simulink model "sampleModel1433_3"  (R2023a)
settings: Solver=VariableStepAuto  StartTime=0.0  StopTime=10.0  RelTol=1e-3
libraries: hdlsllib x7, simulink x2
settings Model: Creator=user1  LastModifiedBy=user1

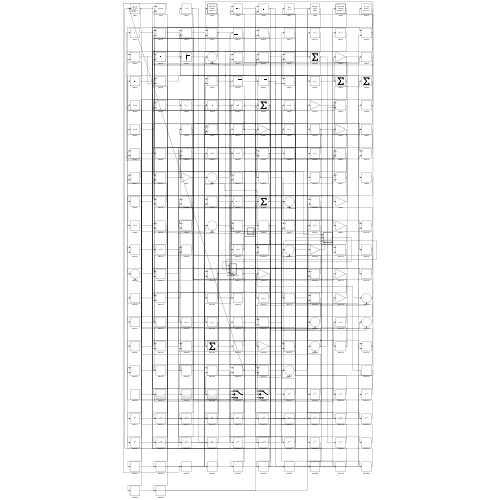
[thumbnail: Simulink's stored preview of the top-level diagram]
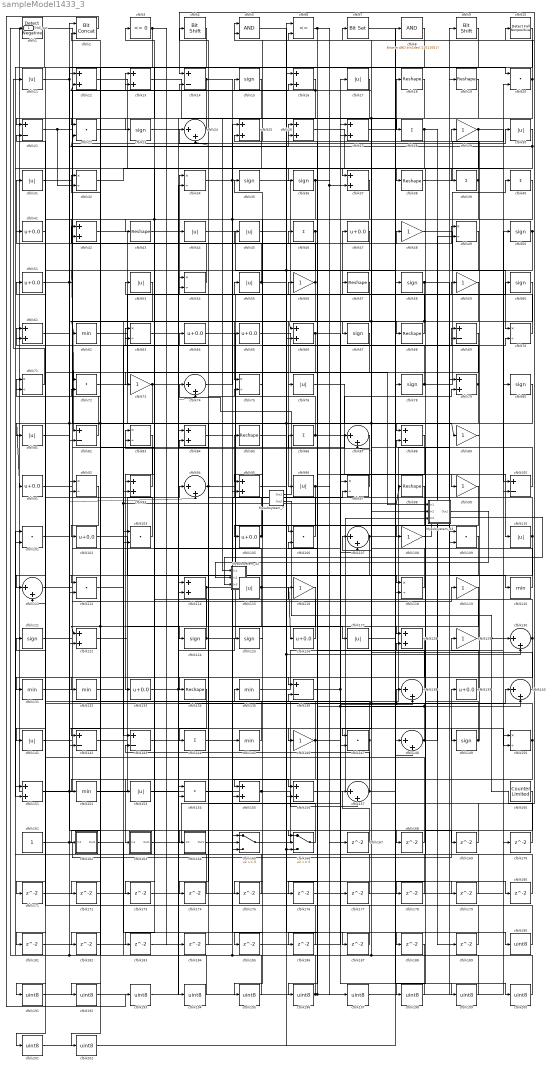
== system sampleModel1433_3 ==
  Mysubsystem_42 : Subsystem  TreatAsAtomicUnit=on  RTWFcnName=Mysubsystem_42
      settings: RTWFcnNameOpts=User specified  RTWFileNameOpts=Use function name
  Mysubsystem_43 : Subsystem  TreatAsAtomicUnit=on  RTWFcnName=Mysubsystem_43
      settings: RTWFcnNameOpts=User specified  RTWFileNameOpts=Use function name
  Mysubsystem_7 : Subsystem  TreatAsAtomicUnit=on  RTWFcnName=Mysubsystem_7
      settings: RTWFcnNameOpts=User specified  RTWFileNameOpts=Use function name
  cfblk1 : hdlsllib/Logic and Bit Operations/Detect Fall Negative  vinit=0  OutDataTypeStr=uint8
  cfblk10 : hdlsllib/Logic and Bit Operations/Detect Fall Nonpositive  vinit=0  OutDataTypeStr=uint8
  cfblk{14,21,69,82,100,136,142..143} (8 alike) : Sum  Inputs=+-  OutDataTypeStr=uint8
  cfblk{20,22,72,101,103,106,109,112,147,154} (10 alike) : DotProduct  OutDataTypeStr=uint8
  cfblk{41,47,51,64..65,91,102,105,126,133,139} (11 alike) : Bias  Bias=0.0  SaturateOnIntegerOverflow=off
  cfblk{24,74,87,94,107,111,130,138,140,148,157} (11 alike) : Sum  Inputs=|++  OutDataTypeStr=uint8
  cfblk{29,48,56,59,73,89,99,108,116,119,129,146} (12 alike) : Gain  OutDataTypeStr=uint8
  cfblk{11,17,30..31,44..45,53,55,76,81,96,110,115,127,141,153} (16 alike) : Abs  OutDataTypeStr=uint8  SaturateOnIntegerOverflow=off
  cfblk{12..13,16,25..27,37,42,61,66,79,84,88,93,95,114,122,128,151,155..156} (21 alike) : Sum  OutDataTypeStr=uint8
  cfblk{32,34,49,54,63,70..71,75,83,92,97,118,150} (13 alike) : Product  Inputs=*/  OutDataTypeStr=uint8  RndMeth=Zero  SaturateOnIntegerOverflow=on
  cfblk{62,120,131..132,135,145,152} (7 alike) : MinMax  OutDataTypeStr=uint8
  cfblk{15,23,35..36,50,58,60,67,78,80,121,124..125,149} (14 alike) : Signum
  cfblk{18..19,38,43,57,68,85,98,134} (9 alike) : Reshape
  cfblk{28,39..40,46,86,144} (6 alike) : Sum  Inputs=+  OutDataTypeStr=uint8
  cfblk160 : hdlsllib/Sources/Counter Limited  uplimit=7  tsamp=-1
  cfblk161 : Constant  OutDataTypeStr=uint8  SampleTime=-1
  cfblk162 : Subsystem
      settings: LibrarySourceBlock=|
      | hdlsllib/Ports &
      | Subsystems/Subsystem
  cfblk163 : Subsystem
      settings: LibrarySourceBlock=|
      | hdlsllib/Ports &
      | Subsystems/Subsystem
  cfblk164 : Subsystem
      settings: LibrarySourceBlock=|
      | hdlsllib/Ports &
      | Subsystems/Subsystem
  cfblk165 : Switch  OutDataTypeStr=uint8  SaturateOnIntegerOverflow=off  InputSameDT=off
  cfblk166 : Switch  OutDataTypeStr=uint8  SaturateOnIntegerOverflow=off  InputSameDT=off
  cfblk{167..189} (23 alike) : Delay  SampleTime=1
  cfblk{190..202} (13 alike) : DataTypeConversion  OutDataTypeStr=uint8  SaturateOnIntegerOverflow=off  RndMeth=Floor
  cfblk2 : hdlsllib/Logic and Bit Operations/Bit Concat  numInputs=2
  cfblk3 : hdlsllib/Logic and Bit Operations/Compare To Zero  relop=<=  OutDataTypeStr=uint8
  cfblk4 : hdlsllib/Logic and Bit Operations/Bit Shift  mode=Shift Left Logical  N=0
  cfblk5 : Logic  AllPortsSameDT=off  OutDataTypeStr=boolean
  cfblk6 : RelationalOperator  Operator=<=  OutDataTypeStr=boolean  InputSameDT=off
  cfblk7 : simulink/Logic and Bit Operations/Bit Set  iBit=0
      settings: LibrarySourceBlock=|
      | hdlsllib/Logic and Bit
      | Operations/Bit Set
  cfblk8 : simulink/Logic and Bit Operations/Bitwise Operator  logicop=AND  UseBitMask=on  BitMask=bin2dec('11011001')  BitMaskRealWorld=Stored Integer
      settings: LibrarySourceBlock=|
      | hdlsllib/Logic and Bit
      | Operations/Bitwise
      | Operator
  cfblk9 : hdlsllib/Logic and Bit Operations/Bit Shift  mode=Shift Left Logical  N=0
  Hdl_out : Outport  OutDataTypeStr=uint8
  wires:
  cfblk105/1 -> cfblk61/1, cfblk75/2
  cfblk73/1 -> cfblk91/1, cfblk172/1, cfblk60/1
  cfblk71/1 -> cfblk11/1
  cfblk145/1 -> cfblk135/1
  cfblk115/1 -> cfblk126/1, cfblk63/2, cfblk174/1
  cfblk131/1 -> cfblk48/1
  cfblk133/1 -> cfblk74/2, cfblk169/1
  cfblk54/1 -> cfblk34/1
  cfblk152/1 -> cfblk94/1
  cfblk86/1 -> cfblk110/1, cfblk54/2
  cfblk1/1 -> cfblk88/1, cfblk101/2
  cfblk31/1 -> cfblk16/2
  cfblk89/1 -> cfblk29/1
  cfblk6/1 -> cfblk37/2, cfblk167/1, cfblk106/1
  cfblk135/1 -> cfblk50/1
  cfblk60/1 -> cfblk96/1
  cfblk118/1 -> cfblk55/1
  cfblk42/1 -> cfblk76/1
  cfblk161/1 -> cfblk139/1, cfblk94/2
  cfblk74/1 -> cfblk25/1
  cfblk49/1 -> cfblk141/1
  cfblk51/1 -> cfblk15/1, cfblk65/1
  cfblk68/1 -> cfblk66/1, cfblk3/1
  cfblk45/1 -> cfblk130/2, cfblk188/1
  cfblk120/1 -> cfblk53/1
  cfblk24/1 -> cfblk21/1
  cfblk35/1 -> cfblk68/1
  cfblk157/1 -> cfblk13/1, cfblk69/2
  cfblk12/1 -> cfblk100/1
  cfblk78/1 -> cfblk40/1, cfblk45/1
  cfblk8/1 -> cfblk202/1
  cfblk160/1 -> cfblk198/1
  cfblk26/1 -> cfblk38/1
  cfblk163/1(Out1) -> cfblk17/1
  cfblk121/1 -> cfblk119/1
  cfblk126/1 -> cfblk83/1
  cfblk141/1 -> cfblk30/1
  cfblk4/1 -> cfblk111/1
  cfblk83/1 -> cfblk133/1
  cfblk25/1 -> cfblk43/1
  cfblk79/1 -> cfblk122/2, cfblk111/2, cfblk26/1
  cfblk124/1 -> cfblk47/1, cfblk42/2
  cfblk96/1 -> cfblk156/2, cfblk177/1
  cfblk37/1 -> cfblk82/1, cfblk73/1, cfblk95/2
  cfblk107/1 -> cfblk115/1, cfblk150/2
  cfblk155/1 -> cfblk157/2, Hdl_out/1
  cfblk20/1 -> Mysubsystem_42/1(In1), cfblk5/1
  cfblk130/1 -> cfblk132/1, cfblk63/1
  cfblk22/1 -> cfblk58/1
  cfblk9/1 -> cfblk23/1
  cfblk50/1 -> cfblk72/1, cfblk166/2, cfblk10/1
  cfblk91/1 -> cfblk79/2
  cfblk103/1 -> cfblk51/1
  cfblk142/1 -> cfblk9/1
  cfblk30/1 -> cfblk128/1, cfblk22/2
  cfblk58/1 -> cfblk62/1, cfblk87/2, cfblk120/1
  cfblk72/1 -> cfblk27/2
  cfblk44/1 -> cfblk78/1
  cfblk18/1 -> cfblk67/1, cfblk36/1
  cfblk27/1 -> cfblk18/1
  cfblk138/1 -> cfblk46/1
  cfblk88/1 -> cfblk136/1
  cfblk153/1 -> cfblk140/1
  cfblk21/1 -> cfblk143/1, cfblk32/2
  cfblk82/1 -> cfblk71/1
  cfblk147/1 -> cfblk4/1, cfblk182/1
  cfblk102/1 -> cfblk148/2
  cfblk165/1 -> cfblk87/1
  cfblk140/1 -> cfblk107/1
  cfblk64/1 -> cfblk118/1
  cfblk19/1 -> cfblk196/1
  cfblk56/1 -> cfblk31/1, cfblk142/1
  cfblk16/1 -> cfblk12/2, cfblk112/2
  cfblk13/1 -> cfblk28/1
  cfblk92/1 -> cfblk102/1
  cfblk129/1 -> cfblk24/1
  cfblk139/1 -> cfblk129/1
  cfblk40/1 -> cfblk105/1
  cfblk134/1 -> cfblk144/1
  cfblk66/1 -> cfblk99/1, cfblk81/1
  cfblk10/1 -> cfblk82/2
  cfblk106/1 -> cfblk35/1
  cfblk94/1 -> cfblk24/2, cfblk147/2
  cfblk164/1(Out1) -> cfblk97/2
  cfblk136/1 -> cfblk140/2, cfblk199/1, cfblk70/2
  cfblk122/1 -> cfblk124/1
  cfblk101/1 -> cfblk164/1(In1)
  cfblk23/1 -> cfblk66/2
  cfblk39/1 -> cfblk5/2, cfblk181/1
  cfblk61/1 -> cfblk146/1
  cfblk149/1 -> cfblk59/1, cfblk128/2
  cfblk93/1 -> cfblk42/1
  cfblk62/1 -> cfblk107/2
  cfblk34/1 -> cfblk127/1, cfblk39/1
  cfblk111/1 -> cfblk49/1
  cfblk3/1 -> cfblk184/1, cfblk192/1
  cfblk47/1 -> cfblk93/1
  cfblk84/1 -> cfblk145/1
  cfblk100/1 -> cfblk6/2
  cfblk53/1 -> cfblk93/2
  cfblk76/1 -> cfblk109/1
  cfblk11/1 -> cfblk20/1, cfblk165/3
  cfblk15/1 -> cfblk114/2
  cfblk48/1 -> cfblk70/1
  cfblk143/1 -> cfblk125/1
  cfblk17/1 -> cfblk92/2
  cfblk46/1 -> cfblk153/1, cfblk186/1
  cfblk70/1 -> cfblk44/1
  cfblk14/1 -> cfblk118/2, cfblk22/1
  cfblk55/1 -> cfblk89/1, cfblk179/1, cfblk32/1
  cfblk81/1 -> cfblk14/2
  cfblk36/1 -> cfblk131/1, cfblk197/1
  cfblk144/1 -> cfblk166/1
  cfblk95/1 -> cfblk108/1
  cfblk166/1 -> cfblk54/1
  cfblk7/1 -> cfblk200/1
  cfblk38/1 -> cfblk20/2
  cfblk148/1 -> cfblk56/1, cfblk138/1, cfblk116/1, cfblk49/2
  cfblk43/1 -> cfblk149/1
  cfblk112/1 -> cfblk86/1, cfblk98/1
  cfblk150/1 -> Mysubsystem_43/2(In2), cfblk121/1, cfblk175/1
  cfblk87/1 -> cfblk83/2
  cfblk110/1 -> cfblk85/1, cfblk142/2
  cfblk97/1 -> cfblk64/1
  cfblk28/1 -> cfblk151/2, cfblk189/1
  cfblk146/1 -> cfblk163/1(In1), cfblk41/1, cfblk138/2
  cfblk125/1 -> cfblk155/1
  cfblk151/1 -> cfblk84/1, cfblk26/2
  cfblk59/1 -> cfblk75/1
  cfblk116/1 -> cfblk122/1, cfblk162/1(In1)
  cfblk85/1 -> cfblk109/2
  cfblk32/1 -> cfblk37/1
  cfblk57/1 -> cfblk112/1
  cfblk29/1 -> cfblk80/1, cfblk183/1
  cfblk80/1 -> cfblk134/1, cfblk147/1
  cfblk132/1 -> cfblk69/1
  cfblk67/1 -> cfblk95/1
  cfblk114/1 -> cfblk152/1, cfblk156/1
  cfblk167/1 -> cfblk157/1
  cfblk5/1 -> cfblk168/1
  cfblk168/1 -> cfblk71/2
  cfblk169/1 -> cfblk16/1
  cfblk170/1 -> cfblk25/2
  cfblk128/1 -> cfblk171/1
  cfblk171/1 -> cfblk165/1
  cfblk172/1 -> cfblk148/1
  cfblk109/1 -> cfblk173/1
  cfblk173/1 -> cfblk79/1
  cfblk174/1 -> cfblk13/2
  cfblk175/1 -> cfblk151/1
  cfblk119/1 -> cfblk176/1
  cfblk176/1 -> cfblk100/2
  cfblk177/1 -> cfblk114/1
  cfblk99/1 -> cfblk178/1
  cfblk178/1 -> cfblk61/2
  cfblk179/1 -> cfblk143/2
  cfblk127/1 -> cfblk180/1
  cfblk180/1 -> cfblk88/2
  cfblk181/1 -> cfblk34/2
  cfblk182/1 -> cfblk103/2
  cfblk183/1 -> cfblk155/2
  cfblk184/1 -> cfblk84/2
  cfblk98/1 -> cfblk185/1
  cfblk185/1 -> cfblk27/1
  cfblk186/1 -> cfblk72/2
  cfblk162/1(Out1) -> cfblk187/1
  cfblk187/1 -> cfblk136/2
  cfblk188/1 -> cfblk1/1
  cfblk189/1 -> cfblk21/2
  cfblk154/1 -> cfblk190/1
  cfblk190/1 -> cfblk97/1
  cfblk69/1 -> cfblk191/1
  cfblk191/1 -> cfblk154/1
  cfblk192/1 -> cfblk154/2
  cfblk2/1 -> cfblk193/1
  cfblk193/1 -> cfblk170/1
  cfblk63/1 -> cfblk194/1
  cfblk194/1 -> cfblk2/1
  cfblk75/1 -> cfblk195/1
  cfblk195/1 -> cfblk2/2
  cfblk196/1 -> cfblk106/2, cfblk150/1, cfblk165/2, cfblk92/1
  cfblk197/1 -> cfblk19/1
  cfblk198/1 -> cfblk101/1, cfblk12/1
  cfblk199/1 -> cfblk7/1
  cfblk200/1 -> cfblk57/1, cfblk103/1
  cfblk41/1 -> cfblk201/1
  cfblk201/1 -> cfblk8/1
  cfblk202/1 -> cfblk166/3, cfblk6/1
  Mysubsystem_7/2(Out2) -> cfblk14/1, cfblk130/1
  Mysubsystem_7/1(Out1) -> cfblk74/1
  cfblk108/1 -> Mysubsystem_42/3(In3)
  cfblk65/1 -> Mysubsystem_43/1(In1)
  cfblk156/1 -> Mysubsystem_43/3(In3)
  Mysubsystem_43/1(Out1) -> Mysubsystem_42/2(In2)

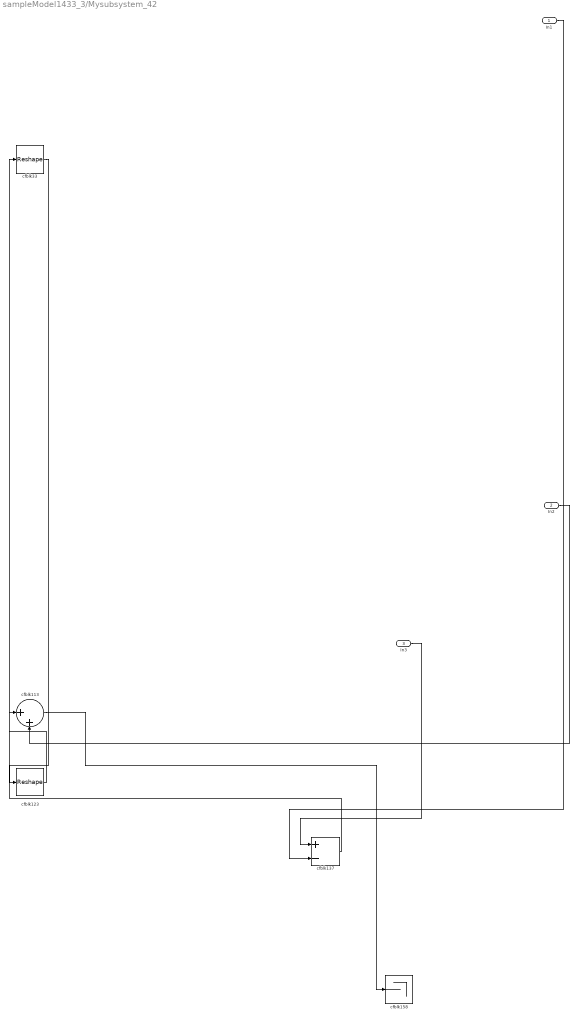
== system sampleModel1433_3/Mysubsystem_42 ==
  In1 : Inport
  In2 : Inport  Port=2
  In3 : Inport  Port=3
  cfblk113 : Sum  Inputs=|++
  cfblk123 : Reshape
  cfblk137 : Sum  Inputs=+-
  cfblk158 : Terminator
  cfblk33 : Reshape
  wires:
  cfblk123/1 -> cfblk113/1
  In3/1 -> cfblk137/1
  cfblk137/1 -> cfblk33/1
  In2/1 -> cfblk113/2
  In1/1 -> cfblk137/2
  cfblk33/1 -> cfblk123/1
  cfblk113/1 -> cfblk158/1

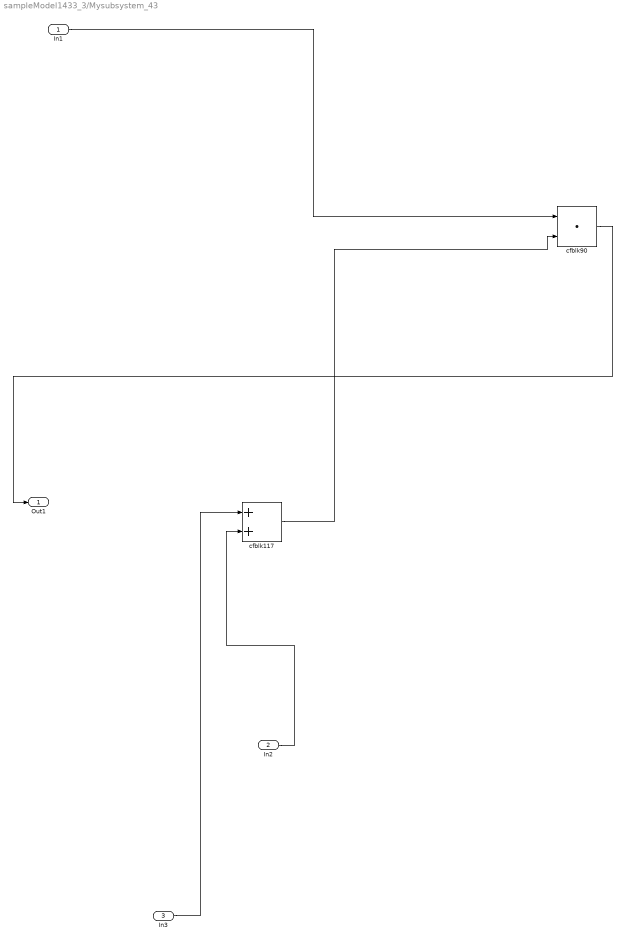
== system sampleModel1433_3/Mysubsystem_43 ==
  In1 : Inport
  In2 : Inport  Port=2
  In3 : Inport  Port=3
  cfblk117 : Sum
  cfblk90 : DotProduct  OutDataTypeStr=Inherit: Inherit via internal rule
  Out1 : Outport
  wires:
  cfblk117/1 -> cfblk90/2
  In3/1 -> cfblk117/1
  cfblk90/1 -> Out1/1
  In1/1 -> cfblk90/1
  In2/1 -> cfblk117/2

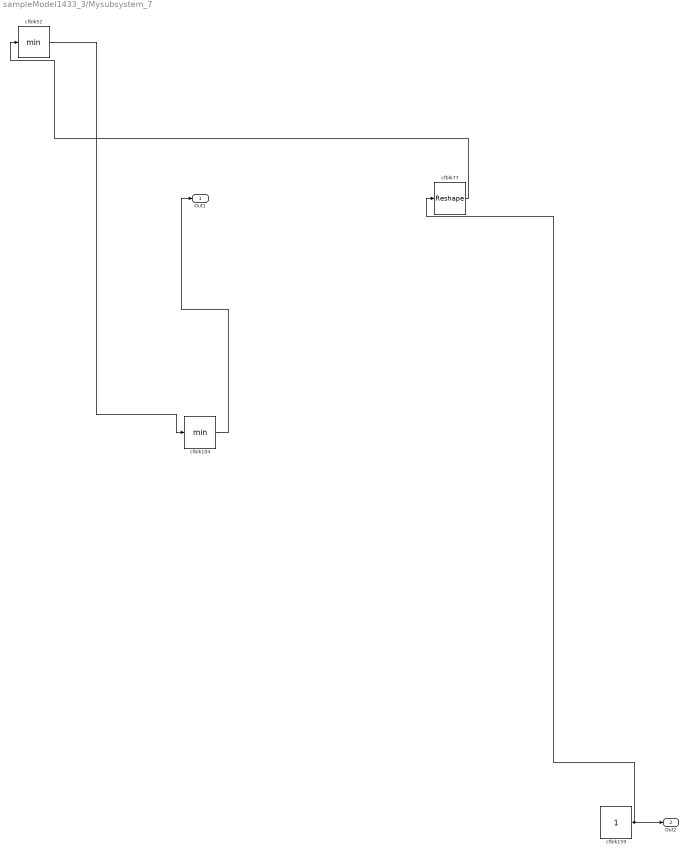
== system sampleModel1433_3/Mysubsystem_7 ==
  cfblk104 : MinMax
  cfblk159 : Constant  SampleTime=-1
  cfblk52 : MinMax
  cfblk77 : Reshape
  Out1 : Outport
  Out2 : Outport  Port=2
  wires:
  cfblk77/1 -> cfblk52/1
  cfblk52/1 -> cfblk104/1
  cfblk159/1 -> Out2/1, cfblk77/1
  cfblk104/1 -> Out1/1

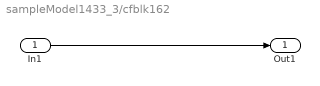
== system sampleModel1433_3/cfblk162 ==
  In1 : Inport
  Out1 : Outport
  wires:
  In1/1 -> Out1/1

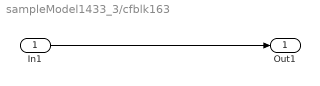
== system sampleModel1433_3/cfblk163 ==
  In1 : Inport
  Out1 : Outport
  wires:
  In1/1 -> Out1/1

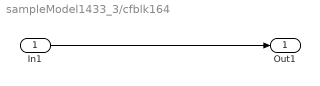
== system sampleModel1433_3/cfblk164 ==
  In1 : Inport
  Out1 : Outport
  wires:
  In1/1 -> Out1/1
